simulink model "ysw3_13"  (R2014a)
settings: Solver=ode45  StartTime=0.0  StopTime=10.0  RelTol=1e-3
settings Model: Creator=Administrator  LastModifiedBy=Administrator

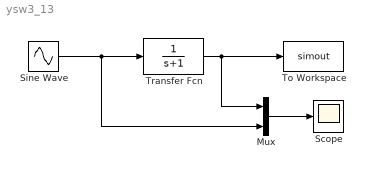
== system ysw3_13 ==
  Mux : Mux  Inputs=2
  Scope : Scope
      settings: TimeRange=10
  Sine Wave : Sin  SampleTime=0
  To Workspace : ToWorkspace  VariableName=simout  SaveFormat=Timeseries  SampleTime=-1
  Transfer Fcn : TransferFcn  Denominator=[1 1]
  wires:
  Transfer Fcn/1 -> Mux/1, To Workspace/1
  Mux/1 -> Scope/1
  Sine Wave/1 -> Mux/2, Transfer Fcn/1
